simulink model "test_mdl"  (R2018a)
settings: Solver=VariableStepAuto  StartTime=0.0  StopTime=10.0  RelTol=1e-3
(part 6 of 8)

== system test_mdl/FD1_CAN_P702_GASD_MY21_DCV_V06/IPMA_ADAS/PARSEDPhysSODLtoGWM_ECG ==
  PARSEDPhysSODLtoGWM_ECG : Constant
  bus_creator : BusCreator  Inputs=1
  port : Outport
  wires:
  bus_creator/1 -> port/1  "PARSEDPhysSODLtoGWM_ECG"
  PARSEDPhysSODLtoGWM_ECG/1 -> bus_creator/1  "PARSEDPhysSODLtoGWM_ECG"

== system test_mdl/FD1_CAN_P702_GASD_MY21_DCV_V06/IPMA_ADAS/PARSEDPhysSODRtoGWM_ECG ==
  PARSEDPhysSODRtoGWM_ECG : Constant
  bus_creator : BusCreator  Inputs=1
  port : Outport
  wires:
  bus_creator/1 -> port/1  "PARSEDPhysSODRtoGWM_ECG"
  PARSEDPhysSODRtoGWM_ECG/1 -> bus_creator/1  "PARSEDPhysSODRtoGWM_ECG"

== system test_mdl/FD1_CAN_P702_GASD_MY21_DCV_V06/IPMA_ADAS/PARSEDPushCCMtoGWM_ECG ==
  PARSEDPhysCCM2toGWM_ECG : Constant
  bus_creator : BusCreator  Inputs=1
  port : Outport
  wires:
  bus_creator/1 -> port/1  "PARSEDPushCCMtoGWM_ECG"
  PARSEDPhysCCM2toGWM_ECG/1 -> bus_creator/1  "PARSEDPhysCCM2toGWM_ECG"

== system test_mdl/FD1_CAN_P702_GASD_MY21_DCV_V06/IPMA_ADAS/PARSEDPushIPMAtoGWM_ECG ==
  PARSEDPhysIPMA2toGWM_ECG : Constant
  bus_creator : BusCreator  Inputs=1
  port : Outport
  wires:
  bus_creator/1 -> port/1  "PARSEDPushIPMAtoGWM_ECG"
  PARSEDPhysIPMA2toGWM_ECG/1 -> bus_creator/1  "PARSEDPhysIPMA2toGWM_ECG"

== system test_mdl/FD1_CAN_P702_GASD_MY21_DCV_V06/IPMA_ADAS/PARSEDPushSODCMCtoGWM ==
  PARSEDPhysSODCMC2toGWM_ECG : Constant
  bus_creator : BusCreator  Inputs=1
  port : Outport
  wires:
  bus_creator/1 -> port/1  "PARSEDPushSODCMCtoGWM"
  PARSEDPhysSODCMC2toGWM_ECG/1 -> bus_creator/1  "PARSEDPhysSODCMC2toGWM_ECG"

== system test_mdl/FD1_CAN_P702_GASD_MY21_DCV_V06/IPMA_ADAS/PARSEDPushSODCMDtoGWM ==
  PARSEDPhysSODCMD2toGWM_ECG : Constant
  bus_creator : BusCreator  Inputs=1
  port : Outport
  wires:
  bus_creator/1 -> port/1  "PARSEDPushSODCMDtoGWM"
  PARSEDPhysSODCMD2toGWM_ECG/1 -> bus_creator/1  "PARSEDPhysSODCMD2toGWM_ECG"

== system test_mdl/FD1_CAN_P702_GASD_MY21_DCV_V06/IPMA_ADAS/PARSEDPushSODLtoGWM_ECG ==
  PARSEDPhysSODL2toGWM_ECG : Constant
  bus_creator : BusCreator  Inputs=1
  port : Outport
  wires:
  bus_creator/1 -> port/1  "PARSEDPushSODLtoGWM_ECG"
  PARSEDPhysSODL2toGWM_ECG/1 -> bus_creator/1  "PARSEDPhysSODL2toGWM_ECG"

== system test_mdl/FD1_CAN_P702_GASD_MY21_DCV_V06/IPMA_ADAS/PARSEDPushSODRtoGWM_ECG ==
  PARSEDPhysSODR2toGWM_ECG : Constant
  bus_creator : BusCreator  Inputs=1
  port : Outport
  wires:
  bus_creator/1 -> port/1  "PARSEDPushSODRtoGWM_ECG"
  PARSEDPhysSODR2toGWM_ECG/1 -> bus_creator/1  "PARSEDPhysSODR2toGWM_ECG"

== system test_mdl/FD1_CAN_P702_GASD_MY21_DCV_V06/IPMA_ADAS/ParkAid_Aud_Warn_Stat ==
  ApaActvSd_D_Actl : Constant
  ApaMde_D_Avail : Constant
  ApaMde_D_Stat : Constant
  FpaChime_D_Rq : Constant
  PrkAidAudioMute_B_Rq : Constant
  PrkAidMsgTxt_D_Rq : Constant
  PrkAidSnsFlCntr_D_Stat : Constant
  PrkAidSnsFlCrnr_D_Stat : Constant
  PrkAidSnsFrCntr_D_Stat : Constant
  PrkAidSnsFrCrnr_D_Stat : Constant
  PrkAidSwtch_B_Stat : Constant
  PrkBrkEl_B_RqFap : Constant
  RpaChime_D_Rq : Constant
  SidePrkSnsL1_D_Stat : Constant
  SidePrkSnsL2_D_Stat : Constant
  SidePrkSnsR1_D_Stat : Constant
  SidePrkSnsR2_D_Stat : Constant
  bus_creator : BusCreator  Inputs=17
  port : Outport
  wires:
  bus_creator/1 -> port/1  "ParkAid_Aud_Warn_Stat"
  ApaActvSd_D_Actl/1 -> bus_creator/1  "ApaActvSd_D_Actl"
  ApaMde_D_Avail/1 -> bus_creator/2  "ApaMde_D_Avail"
  ApaMde_D_Stat/1 -> bus_creator/3  "ApaMde_D_Stat"
  FpaChime_D_Rq/1 -> bus_creator/4  "FpaChime_D_Rq"
  PrkAidAudioMute_B_Rq/1 -> bus_creator/5  "PrkAidAudioMute_B_Rq"
  PrkAidMsgTxt_D_Rq/1 -> bus_creator/6  "PrkAidMsgTxt_D_Rq"
  PrkAidSnsFlCntr_D_Stat/1 -> bus_creator/7  "PrkAidSnsFlCntr_D_Stat"
  PrkAidSnsFlCrnr_D_Stat/1 -> bus_creator/8  "PrkAidSnsFlCrnr_D_Stat"
  PrkAidSnsFrCntr_D_Stat/1 -> bus_creator/9  "PrkAidSnsFrCntr_D_Stat"
  PrkAidSnsFrCrnr_D_Stat/1 -> bus_creator/10  "PrkAidSnsFrCrnr_D_Stat"
  PrkAidSwtch_B_Stat/1 -> bus_creator/11  "PrkAidSwtch_B_Stat"
  PrkBrkEl_B_RqFap/1 -> bus_creator/12  "PrkBrkEl_B_RqFap"
  RpaChime_D_Rq/1 -> bus_creator/13  "RpaChime_D_Rq"
  SidePrkSnsL1_D_Stat/1 -> bus_creator/14  "SidePrkSnsL1_D_Stat"
  SidePrkSnsL2_D_Stat/1 -> bus_creator/15  "SidePrkSnsL2_D_Stat"
  SidePrkSnsR1_D_Stat/1 -> bus_creator/16  "SidePrkSnsR1_D_Stat"
  SidePrkSnsR2_D_Stat/1 -> bus_creator/17  "SidePrkSnsR2_D_Stat"

== system test_mdl/FD1_CAN_P702_GASD_MY21_DCV_V06/IPMA_ADAS/ParkAid_Aud_Warn_Stat2 ==
  ApaBrk_A_Rq : Constant
  ApaBrk_D_Rq : Constant
  ApaLongCtrlEnbl_D_Rq : Constant
  PrkAidChime_D_Stat : Constant
  PrkAidFront_D_Stat : Constant
  PrkAidLamp_D_Rq : Constant
  PrkAidRear_D_Stat : Constant
  PrkAidSnsRlCntr_D_Stat : Constant
  PrkAidSnsRlCrnr_D_Stat : Constant
  PrkAidSnsRrCntr_D_Stat : Constant
  PrkAidSnsRrCrnr_D_Stat : Constant
  PrkAid_D_Falt : Constant
  SidePrkSnsL3_D_Stat : Constant
  SidePrkSnsL4_D_Stat : Constant
  SidePrkSnsR3_D_Stat : Constant
  SidePrkSnsR4_D_Stat : Constant
  bus_creator : BusCreator  Inputs=16
  port : Outport
  wires:
  bus_creator/1 -> port/1  "ParkAid_Aud_Warn_Stat2"
  ApaBrk_A_Rq/1 -> bus_creator/1  "ApaBrk_A_Rq"
  ApaBrk_D_Rq/1 -> bus_creator/2  "ApaBrk_D_Rq"
  ApaLongCtrlEnbl_D_Rq/1 -> bus_creator/3  "ApaLongCtrlEnbl_D_Rq"
  PrkAidChime_D_Stat/1 -> bus_creator/4  "PrkAidChime_D_Stat"
  PrkAidFront_D_Stat/1 -> bus_creator/5  "PrkAidFront_D_Stat"
  PrkAidLamp_D_Rq/1 -> bus_creator/6  "PrkAidLamp_D_Rq"
  PrkAidRear_D_Stat/1 -> bus_creator/7  "PrkAidRear_D_Stat"
  PrkAidSnsRlCntr_D_Stat/1 -> bus_creator/8  "PrkAidSnsRlCntr_D_Stat"
  PrkAidSnsRlCrnr_D_Stat/1 -> bus_creator/9  "PrkAidSnsRlCrnr_D_Stat"
  PrkAidSnsRrCntr_D_Stat/1 -> bus_creator/10  "PrkAidSnsRrCntr_D_Stat"
  PrkAidSnsRrCrnr_D_Stat/1 -> bus_creator/11  "PrkAidSnsRrCrnr_D_Stat"
  PrkAid_D_Falt/1 -> bus_creator/12  "PrkAid_D_Falt"
  SidePrkSnsL3_D_Stat/1 -> bus_creator/13  "SidePrkSnsL3_D_Stat"
  SidePrkSnsL4_D_Stat/1 -> bus_creator/14  "SidePrkSnsL4_D_Stat"
  SidePrkSnsR3_D_Stat/1 -> bus_creator/15  "SidePrkSnsR3_D_Stat"
  SidePrkSnsR4_D_Stat/1 -> bus_creator/16  "SidePrkSnsR4_D_Stat"

== system test_mdl/FD1_CAN_P702_GASD_MY21_DCV_V06/IPMA_ADAS/ParkAid_Data ==
  ApaAcsy_D_RqDrv : Constant
  ApaActvSide2_D_Stat : Constant
  ApaButtnPrssd_B_Stat : Constant
  ApaChime_D_Rq : Constant
  ApaGearShif_D_RqDrv : Constant
  ApaLongCtl_D_RqDrv : Constant
  ApaMsgTxt_D_Rq : Constant
  ApaScan_D_Stat : Constant
  ApaSelPoa_D_Stat : Constant
  ApaSelPpa_D_Stat : Constant
  ApaSelSapp_D_Stat : Constant
  ApaSteScanMde_D_Stat : Constant
  ApaSteWhl_D_RqDrv : Constant
  ApaSys_D_Stat : Constant
  ApaTrgtDist_D_Stat : Constant
  EPASExtAngleStatReq : Constant
  ExtSteeringAngleReq2 : Constant
  SAPPStatusCoding : Constant
  bus_creator : BusCreator  Inputs=18
  port : Outport
  wires:
  bus_creator/1 -> port/1  "ParkAid_Data"
  ApaAcsy_D_RqDrv/1 -> bus_creator/1  "ApaAcsy_D_RqDrv"
  ApaActvSide2_D_Stat/1 -> bus_creator/2  "ApaActvSide2_D_Stat"
  ApaButtnPrssd_B_Stat/1 -> bus_creator/3  "ApaButtnPrssd_B_Stat"
  ApaChime_D_Rq/1 -> bus_creator/4  "ApaChime_D_Rq"
  ApaGearShif_D_RqDrv/1 -> bus_creator/5  "ApaGearShif_D_RqDrv"
  ApaLongCtl_D_RqDrv/1 -> bus_creator/6  "ApaLongCtl_D_RqDrv"
  ApaMsgTxt_D_Rq/1 -> bus_creator/7  "ApaMsgTxt_D_Rq"
  ApaScan_D_Stat/1 -> bus_creator/8  "ApaScan_D_Stat"
  ApaSelPoa_D_Stat/1 -> bus_creator/9  "ApaSelPoa_D_Stat"
  ApaSelPpa_D_Stat/1 -> bus_creator/10  "ApaSelPpa_D_Stat"
  ApaSelSapp_D_Stat/1 -> bus_creator/11  "ApaSelSapp_D_Stat"
  ApaSteScanMde_D_Stat/1 -> bus_creator/12  "ApaSteScanMde_D_Stat"
  ApaSteWhl_D_RqDrv/1 -> bus_creator/13  "ApaSteWhl_D_RqDrv"
  ApaSys_D_Stat/1 -> bus_creator/14  "ApaSys_D_Stat"
  ApaTrgtDist_D_Stat/1 -> bus_creator/15  "ApaTrgtDist_D_Stat"
  EPASExtAngleStatReq/1 -> bus_creator/16  "EPASExtAngleStatReq"
  ExtSteeringAngleReq2/1 -> bus_creator/17  "ExtSteeringAngleReq2"
  SAPPStatusCoding/1 -> bus_creator/18  "SAPPStatusCoding"

== system test_mdl/FD1_CAN_P702_GASD_MY21_DCV_V06/IPMA_ADAS/ParkAid_Data2 ==
  PrkAidAcsyFront_D_Stat : Constant
  PrkAidAcsyRear_D_Stat : Constant
  PrkAidDrvDir_D_Stat : Constant
  PrkAidRdiusLeft_L_Dsply : Constant
  PrkAidRdiusRight_L_Dsply : Constant
  bus_creator : BusCreator  Inputs=5
  port : Outport
  wires:
  bus_creator/1 -> port/1  "ParkAid_Data2"
  PrkAidAcsyFront_D_Stat/1 -> bus_creator/1  "PrkAidAcsyFront_D_Stat"
  PrkAidAcsyRear_D_Stat/1 -> bus_creator/2  "PrkAidAcsyRear_D_Stat"
  PrkAidDrvDir_D_Stat/1 -> bus_creator/3  "PrkAidDrvDir_D_Stat"
  PrkAidRdiusLeft_L_Dsply/1 -> bus_creator/4  "PrkAidRdiusLeft_L_Dsply"
  PrkAidRdiusRight_L_Dsply/1 -> bus_creator/5  "PrkAidRdiusRight_L_Dsply"

== system test_mdl/FD1_CAN_P702_GASD_MY21_DCV_V06/IPMA_ADAS/ParkAid_Data_2 ==
  FapLcDistToObj_L_Actl : Constant
  TrnRngDRqFap_No_Cnt : Constant
  TrnRngDRqFap_No_Cs : Constant
  TrnRng_D_RqFap : Constant
  Veh_V_RqFap : Constant
  bus_creator : BusCreator  Inputs=5
  port : Outport
  wires:
  bus_creator/1 -> port/1  "ParkAid_Data_2"
  FapLcDistToObj_L_Actl/1 -> bus_creator/1  "FapLcDistToObj_L_Actl"
  TrnRngDRqFap_No_Cnt/1 -> bus_creator/2  "TrnRngDRqFap_No_Cnt"
  TrnRngDRqFap_No_Cs/1 -> bus_creator/3  "TrnRngDRqFap_No_Cs"
  TrnRng_D_RqFap/1 -> bus_creator/4  "TrnRng_D_RqFap"
  Veh_V_RqFap/1 -> bus_creator/5  "Veh_V_RqFap"

== system test_mdl/FD1_CAN_P702_GASD_MY21_DCV_V06/IPMA_ADAS/Personality_CCM_Data ==
  FeatConfigCcmActl : Constant
  FeatNoCcmActl : Constant
  PersIndexCcm_D_Actl : Constant
  bus_creator : BusCreator  Inputs=3
  port : Outport
  wires:
  bus_creator/1 -> port/1  "Personality_CCM_Data"
  FeatConfigCcmActl/1 -> bus_creator/1  "FeatConfigCcmActl"
  FeatNoCcmActl/1 -> bus_creator/2  "FeatNoCcmActl"
  PersIndexCcm_D_Actl/1 -> bus_creator/3  "PersIndexCcm_D_Actl"

== system test_mdl/FD1_CAN_P702_GASD_MY21_DCV_V06/IPMA_ADAS/Personality_IPMB_Data ==
  FeatConfigIpmbActl : Constant
  FeatNoIpmbActl : Constant
  PersIndexIpmb_D_Actl : Constant
  bus_creator : BusCreator  Inputs=3
  port : Outport
  wires:
  bus_creator/1 -> port/1  "Personality_IPMB_Data"
  FeatConfigIpmbActl/1 -> bus_creator/1  "FeatConfigIpmbActl"
  FeatNoIpmbActl/1 -> bus_creator/2  "FeatNoIpmbActl"
  PersIndexIpmb_D_Actl/1 -> bus_creator/3  "PersIndexIpmb_D_Actl"

== system test_mdl/FD1_CAN_P702_GASD_MY21_DCV_V06/IPMA_ADAS/Side_Detect_L_Stat ==
  BttLeft_D_RqDrv : Constant
  BttLeft_D_Stat : Constant
  CtaAlrtLeft2_D_Stat : Constant
  CtaAlrtLeft_D_Stat : Constant
  CtaBrkLeftMsgTxt_B_Rq : Constant
  CtaLeftBrkDecel_B_Rq : Constant
  CtaLeftBrkEnbl_B_Rq : Constant
  CtaLeft_D_Stat : Constant
  CtaSnsLeft_D_Stat : Constant
  Side_Detect_L_Illum : Constant
  SodAlrtLeft_D_Stat : Constant
  SodDetctLeft_D_Stat : Constant
  SodLeft_D_Stat : Constant
  SodSnsLeft_D_Stat : Constant
  SodWarnLeft_Prd_Rq : Constant
  bus_creator : BusCreator  Inputs=15
  port : Outport
  wires:
  bus_creator/1 -> port/1  "Side_Detect_L_Stat"
  BttLeft_D_RqDrv/1 -> bus_creator/1  "BttLeft_D_RqDrv"
  BttLeft_D_Stat/1 -> bus_creator/2  "BttLeft_D_Stat"
  CtaAlrtLeft2_D_Stat/1 -> bus_creator/3  "CtaAlrtLeft2_D_Stat"
  CtaAlrtLeft_D_Stat/1 -> bus_creator/4  "CtaAlrtLeft_D_Stat"
  CtaBrkLeftMsgTxt_B_Rq/1 -> bus_creator/5  "CtaBrkLeftMsgTxt_B_Rq"
  CtaLeftBrkDecel_B_Rq/1 -> bus_creator/6  "CtaLeftBrkDecel_B_Rq"
  CtaLeftBrkEnbl_B_Rq/1 -> bus_creator/7  "CtaLeftBrkEnbl_B_Rq"
  CtaLeft_D_Stat/1 -> bus_creator/8  "CtaLeft_D_Stat"
  CtaSnsLeft_D_Stat/1 -> bus_creator/9  "CtaSnsLeft_D_Stat"
  Side_Detect_L_Illum/1 -> bus_creator/10  "Side_Detect_L_Illum"
  SodAlrtLeft_D_Stat/1 -> bus_creator/11  "SodAlrtLeft_D_Stat"
  SodDetctLeft_D_Stat/1 -> bus_creator/12  "SodDetctLeft_D_Stat"
  SodLeft_D_Stat/1 -> bus_creator/13  "SodLeft_D_Stat"
  SodSnsLeft_D_Stat/1 -> bus_creator/14  "SodSnsLeft_D_Stat"
  SodWarnLeft_Prd_Rq/1 -> bus_creator/15  "SodWarnLeft_Prd_Rq"

== system test_mdl/FD1_CAN_P702_GASD_MY21_DCV_V06/IPMA_ADAS/Side_Detect_R_Stat ==
  BttRight_D_RqDrv : Constant
  BttRight_D_Stat : Constant
  CtaAlrtRight2_D_Stat : Constant
  CtaAlrtRight_D_Stat : Constant
  CtaBrkRightMsgTxt_B_Rq : Constant
  CtaRightBrkDecel_B_Rq : Constant
  CtaRightBrkEnbl_B_Rq : Constant
  CtaRight_D_Stat : Constant
  CtaSnsRight_D_Stat : Constant
  Side_Detect_R_Illum : Constant
  SodAlrtRight_D_Stat : Constant
  SodDetctRight_D_Stat : Constant
  SodRight_D_Stat : Constant
  SodSnsRight_D_Stat : Constant
  SodWarnRight_Prd_Rq : Constant
  bus_creator : BusCreator  Inputs=15
  port : Outport
  wires:
  bus_creator/1 -> port/1  "Side_Detect_R_Stat"
  BttRight_D_RqDrv/1 -> bus_creator/1  "BttRight_D_RqDrv"
  BttRight_D_Stat/1 -> bus_creator/2  "BttRight_D_Stat"
  CtaAlrtRight2_D_Stat/1 -> bus_creator/3  "CtaAlrtRight2_D_Stat"
  CtaAlrtRight_D_Stat/1 -> bus_creator/4  "CtaAlrtRight_D_Stat"
  CtaBrkRightMsgTxt_B_Rq/1 -> bus_creator/5  "CtaBrkRightMsgTxt_B_Rq"
  CtaRightBrkDecel_B_Rq/1 -> bus_creator/6  "CtaRightBrkDecel_B_Rq"
  CtaRightBrkEnbl_B_Rq/1 -> bus_creator/7  "CtaRightBrkEnbl_B_Rq"
  CtaRight_D_Stat/1 -> bus_creator/8  "CtaRight_D_Stat"
  CtaSnsRight_D_Stat/1 -> bus_creator/9  "CtaSnsRight_D_Stat"
  Side_Detect_R_Illum/1 -> bus_creator/10  "Side_Detect_R_Illum"
  SodAlrtRight_D_Stat/1 -> bus_creator/11  "SodAlrtRight_D_Stat"
  SodDetctRight_D_Stat/1 -> bus_creator/12  "SodDetctRight_D_Stat"
  SodRight_D_Stat/1 -> bus_creator/13  "SodRight_D_Stat"
  SodSnsRight_D_Stat/1 -> bus_creator/14  "SodSnsRight_D_Stat"
  SodWarnRight_Prd_Rq/1 -> bus_creator/15  "SodWarnRight_Prd_Rq"

== system test_mdl/FD1_CAN_P702_GASD_MY21_DCV_V06/IPMA_ADAS/Steer_Assist_Data ==
  CmbbObjClass_D_Stat : Constant
  CmbbObjColl_T_Actl : Constant
  CmbbObjConfdnc_D_Stat : Constant
  CmbbObjDistLat_L_Actl : Constant
  CmbbObjDistLong_L_Actl : Constant
  CmbbObjRelLat_V_Actl : Constant
  CmbbObjRelLong_V_Actl : Constant
  EsaEnbl_D2_Rq : Constant
  bus_creator : BusCreator  Inputs=8
  port : Outport
  wires:
  bus_creator/1 -> port/1  "Steer_Assist_Data"
  CmbbObjClass_D_Stat/1 -> bus_creator/1  "CmbbObjClass_D_Stat"
  CmbbObjColl_T_Actl/1 -> bus_creator/2  "CmbbObjColl_T_Actl"
  CmbbObjConfdnc_D_Stat/1 -> bus_creator/3  "CmbbObjConfdnc_D_Stat"
  CmbbObjDistLat_L_Actl/1 -> bus_creator/4  "CmbbObjDistLat_L_Actl"
  CmbbObjDistLong_L_Actl/1 -> bus_creator/5  "CmbbObjDistLong_L_Actl"
  CmbbObjRelLat_V_Actl/1 -> bus_creator/6  "CmbbObjRelLat_V_Actl"
  CmbbObjRelLong_V_Actl/1 -> bus_creator/7  "CmbbObjRelLong_V_Actl"
  EsaEnbl_D2_Rq/1 -> bus_creator/8  "EsaEnbl_D2_Rq"

== system test_mdl/FD1_CAN_P702_GASD_MY21_DCV_V06/IPMA_ADAS/SuspensionRoad_Data ==
  SrpDistLeft_L_Actl : Constant
  SrpDistRight_L_Actl : Constant
  SrpEventLeft_D_Stat : Constant
  SrpEventRight_D_Stat : Constant
  SrpHghtLeft_L_Actl : Constant
  SrpHghtRight_L_Actl : Constant
  SrpSigValid_B_Stat : Constant
  SuspClkSync_No_Actl : Constant
  bus_creator : BusCreator  Inputs=8
  port : Outport
  wires:
  bus_creator/1 -> port/1  "SuspensionRoad_Data"
  SrpDistLeft_L_Actl/1 -> bus_creator/1  "SrpDistLeft_L_Actl"
  SrpDistRight_L_Actl/1 -> bus_creator/2  "SrpDistRight_L_Actl"
  SrpEventLeft_D_Stat/1 -> bus_creator/3  "SrpEventLeft_D_Stat"
  SrpEventRight_D_Stat/1 -> bus_creator/4  "SrpEventRight_D_Stat"
  SrpHghtLeft_L_Actl/1 -> bus_creator/5  "SrpHghtLeft_L_Actl"
  SrpHghtRight_L_Actl/1 -> bus_creator/6  "SrpHghtRight_L_Actl"
  SrpSigValid_B_Stat/1 -> bus_creator/7  "SrpSigValid_B_Stat"
  SuspClkSync_No_Actl/1 -> bus_creator/8  "SuspClkSync_No_Actl"

== system test_mdl/FD1_CAN_P702_GASD_MY21_DCV_V06/IPMA_ADAS/TesterPhysicalResCCM ==
  TesterPhysicalResCCM : Constant
  bus_creator : BusCreator  Inputs=1
  port : Outport
  wires:
  bus_creator/1 -> port/1  "TesterPhysicalResCCM"
  TesterPhysicalResCCM/1 -> bus_creator/1  "TesterPhysicalResCCM"

== system test_mdl/FD1_CAN_P702_GASD_MY21_DCV_V06/IPMA_ADAS/TesterPhysicalResIPMA ==
  TesterPhysicalResIPMA : Constant
  bus_creator : BusCreator  Inputs=1
  port : Outport
  wires:
  bus_creator/1 -> port/1  "TesterPhysicalResIPMA"
  TesterPhysicalResIPMA/1 -> bus_creator/1  "TesterPhysicalResIPMA"

== system test_mdl/FD1_CAN_P702_GASD_MY21_DCV_V06/IPMA_ADAS/TesterPhysicalResSODCMC ==
  TesterPhysicalResSODCMC : Constant
  bus_creator : BusCreator  Inputs=1
  port : Outport
  wires:
  bus_creator/1 -> port/1  "TesterPhysicalResSODCMC"
  TesterPhysicalResSODCMC/1 -> bus_creator/1  "TesterPhysicalResSODCMC"

== system test_mdl/FD1_CAN_P702_GASD_MY21_DCV_V06/IPMA_ADAS/TesterPhysicalResSODCMD ==
  TesterPhysicalResSODCMD : Constant
  bus_creator : BusCreator  Inputs=1
  port : Outport
  wires:
  bus_creator/1 -> port/1  "TesterPhysicalResSODCMD"
  TesterPhysicalResSODCMD/1 -> bus_creator/1  "TesterPhysicalResSODCMD"

== system test_mdl/FD1_CAN_P702_GASD_MY21_DCV_V06/IPMA_ADAS/TesterPhysicalResSODL ==
  TesterPhysicalResSODL : Constant
  bus_creator : BusCreator  Inputs=1
  port : Outport
  wires:
  bus_creator/1 -> port/1  "TesterPhysicalResSODL"
  TesterPhysicalResSODL/1 -> bus_creator/1  "TesterPhysicalResSODL"

== system test_mdl/FD1_CAN_P702_GASD_MY21_DCV_V06/IPMA_ADAS/TesterPhysicalResSODR ==
  TesterPhysicalResSODR : Constant
  bus_creator : BusCreator  Inputs=1
  port : Outport
  wires:
  bus_creator/1 -> port/1  "TesterPhysicalResSODR"
  TesterPhysicalResSODR/1 -> bus_creator/1  "TesterPhysicalResSODR"

== system test_mdl/FD1_CAN_P702_GASD_MY21_DCV_V06/IPMA_ADAS/Traffic_RecognitnData ==
  TsrMsgTxt_D_Rq : Constant
  TsrOswWarnMsgTxt_D_Rq : Constant
  TsrOvtkMsgTxt2_D_Rq : Constant
  TsrOvtkMsgTxt_D_Rq : Constant
  TsrOvtkStatMsgTxt_D_Rq : Constant
  TsrStatMsgTxt_D_Rq : Constant
  TsrVLim1MsgTxt_D_Rq : Constant
  TsrVLim2MsgTxt_D_Rq : Constant
  TsrVl1PrmntMsgTxt_D_Rq : Constant
  TsrVl1RstrcMsgTxt2_D_Rq : Constant
  TsrVl1RstrcMsgTxt_D_Rq : Constant
  TsrVl1StatMsgTxt_D_Rq : Constant
  TsrVl2PrmntMsgTxt_D_Rq : Constant
  TsrVl2RstrcMsgTxt2_D_Rq : Constant
  TsrVl2RstrcMsgTxt_D_Rq : Constant
  TsrVl2StatMsgTxt_D_Rq : Constant
  TsrVlUnitMsgTxt_D_Rq : Constant
  WwaWarn_B_Rq : Constant
  bus_creator : BusCreator  Inputs=18
  port : Outport
  wires:
  bus_creator/1 -> port/1  "Traffic_RecognitnData"
  TsrMsgTxt_D_Rq/1 -> bus_creator/1  "TsrMsgTxt_D_Rq"
  TsrOswWarnMsgTxt_D_Rq/1 -> bus_creator/2  "TsrOswWarnMsgTxt_D_Rq"
  TsrOvtkMsgTxt2_D_Rq/1 -> bus_creator/3  "TsrOvtkMsgTxt2_D_Rq"
  TsrOvtkMsgTxt_D_Rq/1 -> bus_creator/4  "TsrOvtkMsgTxt_D_Rq"
  TsrOvtkStatMsgTxt_D_Rq/1 -> bus_creator/5  "TsrOvtkStatMsgTxt_D_Rq"
  TsrStatMsgTxt_D_Rq/1 -> bus_creator/6  "TsrStatMsgTxt_D_Rq"
  TsrVLim1MsgTxt_D_Rq/1 -> bus_creator/7  "TsrVLim1MsgTxt_D_Rq"
  TsrVLim2MsgTxt_D_Rq/1 -> bus_creator/8  "TsrVLim2MsgTxt_D_Rq"
  TsrVl1PrmntMsgTxt_D_Rq/1 -> bus_creator/9  "TsrVl1PrmntMsgTxt_D_Rq"
  TsrVl1RstrcMsgTxt2_D_Rq/1 -> bus_creator/10  "TsrVl1RstrcMsgTxt2_D_Rq"
  TsrVl1RstrcMsgTxt_D_Rq/1 -> bus_creator/11  "TsrVl1RstrcMsgTxt_D_Rq"
  TsrVl1StatMsgTxt_D_Rq/1 -> bus_creator/12  "TsrVl1StatMsgTxt_D_Rq"
  TsrVl2PrmntMsgTxt_D_Rq/1 -> bus_creator/13  "TsrVl2PrmntMsgTxt_D_Rq"
  TsrVl2RstrcMsgTxt2_D_Rq/1 -> bus_creator/14  "TsrVl2RstrcMsgTxt2_D_Rq"
  TsrVl2RstrcMsgTxt_D_Rq/1 -> bus_creator/15  "TsrVl2RstrcMsgTxt_D_Rq"
  TsrVl2StatMsgTxt_D_Rq/1 -> bus_creator/16  "TsrVl2StatMsgTxt_D_Rq"
  TsrVlUnitMsgTxt_D_Rq/1 -> bus_creator/17  "TsrVlUnitMsgTxt_D_Rq"
  WwaWarn_B_Rq/1 -> bus_creator/18  "WwaWarn_B_Rq"

== system test_mdl/FD1_CAN_P702_GASD_MY21_DCV_V06/IPMA_ADAS/TrailerAid_Stat3 ==
  HitchToTrlrAxle_L_Calc2 : Constant
  HitchToVehAxle_L_Calc : Constant
  TrlrAidTrgtId_No_Actl : Constant
  TrlrAid_An3_Actl : Constant
  TrlrAid_AnRate2_Actl : Constant
  TrlrAid_D2_Stat : Constant
  TrlrAnCalib_B_Complt : Constant
  TrlrAnOffstDir_D_Calc : Constant
  TrlrAnOffst_An_Calc : Constant
  TrlrRvrse_D_Stat : Constant
  TrlrTrgtAcquire_D_Stat : Constant
  bus_creator : BusCreator  Inputs=11
  port : Outport
  wires:
  bus_creator/1 -> port/1  "TrailerAid_Stat3"
  HitchToTrlrAxle_L_Calc2/1 -> bus_creator/1  "HitchToTrlrAxle_L_Calc2"
  HitchToVehAxle_L_Calc/1 -> bus_creator/2  "HitchToVehAxle_L_Calc"
  TrlrAidTrgtId_No_Actl/1 -> bus_creator/3  "TrlrAidTrgtId_No_Actl"
  TrlrAid_An3_Actl/1 -> bus_creator/4  "TrlrAid_An3_Actl"
  TrlrAid_AnRate2_Actl/1 -> bus_creator/5  "TrlrAid_AnRate2_Actl"
  TrlrAid_D2_Stat/1 -> bus_creator/6  "TrlrAid_D2_Stat"
  TrlrAnCalib_B_Complt/1 -> bus_creator/7  "TrlrAnCalib_B_Complt"
  TrlrAnOffstDir_D_Calc/1 -> bus_creator/8  "TrlrAnOffstDir_D_Calc"
  TrlrAnOffst_An_Calc/1 -> bus_creator/9  "TrlrAnOffst_An_Calc"
  TrlrRvrse_D_Stat/1 -> bus_creator/10  "TrlrRvrse_D_Stat"
  TrlrTrgtAcquire_D_Stat/1 -> bus_creator/11  "TrlrTrgtAcquire_D_Stat"

== system test_mdl/FD1_CAN_P702_GASD_MY21_DCV_V06/PCM/DCACA_Data4 ==
  DcacElPw_D_Stat : Constant
  DcacEngOnMsgTxt_D_Rq : Constant
  DcacFaltMsgTxt_D_Rq : Constant
  DcacGfciTest_B_Rq : Constant
  DcacHw_D_Confg : Constant
  DcacLedCtl_D_Rq : Constant
  DcacLoFuelMsgTxt_D_Rq : Constant
  DcacOn_B_Rq : Constant
  DcacOut1_Pw_Dsply : Constant
  DcacOut2_Pw_Dsply : Constant
  DcacOut_Pw_DsplyMx : Constant
  DcacSys_B_Falt : Constant
  PwBedPnlEnbl_B_Rq : Constant
  bus_creator : BusCreator  Inputs=13
  port : Outport
  wires:
  bus_creator/1 -> port/1  "DCACA_Data4"
  DcacElPw_D_Stat/1 -> bus_creator/1  "DcacElPw_D_Stat"
  DcacEngOnMsgTxt_D_Rq/1 -> bus_creator/2  "DcacEngOnMsgTxt_D_Rq"
  DcacFaltMsgTxt_D_Rq/1 -> bus_creator/3  "DcacFaltMsgTxt_D_Rq"
  DcacGfciTest_B_Rq/1 -> bus_creator/4  "DcacGfciTest_B_Rq"
  DcacHw_D_Confg/1 -> bus_creator/5  "DcacHw_D_Confg"
  DcacLedCtl_D_Rq/1 -> bus_creator/6  "DcacLedCtl_D_Rq"
  DcacLoFuelMsgTxt_D_Rq/1 -> bus_creator/7  "DcacLoFuelMsgTxt_D_Rq"
  DcacOn_B_Rq/1 -> bus_creator/8  "DcacOn_B_Rq"
  DcacOut1_Pw_Dsply/1 -> bus_creator/9  "DcacOut1_Pw_Dsply"
  DcacOut2_Pw_Dsply/1 -> bus_creator/10  "DcacOut2_Pw_Dsply"
  DcacOut_Pw_DsplyMx/1 -> bus_creator/11  "DcacOut_Pw_DsplyMx"
  DcacSys_B_Falt/1 -> bus_creator/12  "DcacSys_B_Falt"
  PwBedPnlEnbl_B_Rq/1 -> bus_creator/13  "PwBedPnlEnbl_B_Rq"

== system test_mdl/FD1_CAN_P702_GASD_MY21_DCV_V06/PCM/EngBrakeData ==
  AccEngStat_D_Actl : Constant
  AccStopMde_D_Rq : Constant
  BPedDrvAppl_D_QF : Constant
  BpedDrvAppl_D_Actl : Constant
  CcMde_D_Actl : Constant
  CcOvrrdActv_B_Actl : Constant
  CcStat_D_Actl : Constant
  CmbbDeny_B_ActlPrpl : Constant
  CmbbEngTqMn_B_Actl : Constant
  EngAout_N_MnAllw : Constant
  PrplTqMnSat_B_Actl : Constant
  Veh_V_DsplyCcSet : Constant
  bus_creator : BusCreator  Inputs=12
  port : Outport
  wires:
  bus_creator/1 -> port/1  "EngBrakeData"
  AccEngStat_D_Actl/1 -> bus_creator/1  "AccEngStat_D_Actl"
  AccStopMde_D_Rq/1 -> bus_creator/2  "AccStopMde_D_Rq"
  BPedDrvAppl_D_QF/1 -> bus_creator/3  "BPedDrvAppl_D_QF"
  BpedDrvAppl_D_Actl/1 -> bus_creator/4  "BpedDrvAppl_D_Actl"
  CcMde_D_Actl/1 -> bus_creator/5  "CcMde_D_Actl"
  CcOvrrdActv_B_Actl/1 -> bus_creator/6  "CcOvrrdActv_B_Actl"
  CcStat_D_Actl/1 -> bus_creator/7  "CcStat_D_Actl"
  CmbbDeny_B_ActlPrpl/1 -> bus_creator/8  "CmbbDeny_B_ActlPrpl"
  CmbbEngTqMn_B_Actl/1 -> bus_creator/9  "CmbbEngTqMn_B_Actl"
  EngAout_N_MnAllw/1 -> bus_creator/10  "EngAout_N_MnAllw"
  PrplTqMnSat_B_Actl/1 -> bus_creator/11  "PrplTqMnSat_B_Actl"
  Veh_V_DsplyCcSet/1 -> bus_creator/12  "Veh_V_DsplyCcSet"

== system test_mdl/FD1_CAN_P702_GASD_MY21_DCV_V06/PCM/EngVehicleSpThrottle ==
  ApedPosPcActl_D_Qf : Constant
  ApedPosPcActl_No_Cnt : Constant
  ApedPosPcActl_No_Cs : Constant
  ApedPos_PcRate_ActlArb : Constant
  ApedPos_Pc_ActlArb : Constant
  EngAout3_N_Actl : Constant
  EngAoutNActl_D_QF : Constant
  EngAout_N_Actl : Constant
  bus_creator : BusCreator  Inputs=8
  port : Outport
  wires:
  bus_creator/1 -> port/1  "EngVehicleSpThrottle"
  ApedPosPcActl_D_Qf/1 -> bus_creator/1  "ApedPosPcActl_D_Qf"
  ApedPosPcActl_No_Cnt/1 -> bus_creator/2  "ApedPosPcActl_No_Cnt"
  ApedPosPcActl_No_Cs/1 -> bus_creator/3  "ApedPosPcActl_No_Cs"
  ApedPos_PcRate_ActlArb/1 -> bus_creator/4  "ApedPos_PcRate_ActlArb"
  ApedPos_Pc_ActlArb/1 -> bus_creator/5  "ApedPos_Pc_ActlArb"
  EngAout3_N_Actl/1 -> bus_creator/6  "EngAout3_N_Actl"
  EngAoutNActl_D_QF/1 -> bus_creator/7  "EngAoutNActl_D_QF"
  EngAout_N_Actl/1 -> bus_creator/8  "EngAout_N_Actl"

== system test_mdl/FD1_CAN_P702_GASD_MY21_DCV_V06/PCM/EngVehicleSpThrottle2 ==
  GearRvrse_D_Actl : Constant
  StrtrMtrCtlMsgTxt_D2_Rq : Constant
  StrtrMtrCtlMsgTxt_D_Rq : Constant
  StrtrMtrDlyStrt_B_Stat : Constant
  VehVActlEng_D_Qf : Constant
  VehVActlEng_No_Cnt : Constant
  VehVActlEng_No_Cs : Constant
  VehVTrlrAid_B_Avail : Constant
  Veh_V_ActlEng : Constant
  Veh_V_RqCcSet : Constant
  bus_creator : BusCreator  Inputs=10
  port : Outport
  wires:
  bus_creator/1 -> port/1  "EngVehicleSpThrottle2"
  GearRvrse_D_Actl/1 -> bus_creator/1  "GearRvrse_D_Actl"
  StrtrMtrCtlMsgTxt_D2_Rq/1 -> bus_creator/2  "StrtrMtrCtlMsgTxt_D2_Rq"
  StrtrMtrCtlMsgTxt_D_Rq/1 -> bus_creator/3  "StrtrMtrCtlMsgTxt_D_Rq"
  StrtrMtrDlyStrt_B_Stat/1 -> bus_creator/4  "StrtrMtrDlyStrt_B_Stat"
  VehVActlEng_D_Qf/1 -> bus_creator/5  "VehVActlEng_D_Qf"
  VehVActlEng_No_Cnt/1 -> bus_creator/6  "VehVActlEng_No_Cnt"
  VehVActlEng_No_Cs/1 -> bus_creator/7  "VehVActlEng_No_Cs"
  VehVTrlrAid_B_Avail/1 -> bus_creator/8  "VehVTrlrAid_B_Avail"
  Veh_V_ActlEng/1 -> bus_creator/9  "Veh_V_ActlEng"
  Veh_V_RqCcSet/1 -> bus_creator/10  "Veh_V_RqCcSet"

== system test_mdl/FD1_CAN_P702_GASD_MY21_DCV_V06/PCM/EngineClimateData ==
  AirAmbTe_D_Qf : Constant
  AirAmb_P_Actl : Constant
  AirAmb_Te_Actl : Constant
  AirAmb_Te_ActlFilt : Constant
  AslChime_B_Rq : Constant
  AslIconDsply_D_Rq : Constant
  DynoMde_B_Cmd : Constant
  EcssLamp_D_RqDsply : Constant
  EngAout_Aa_Actl : Constant
  GasPrtc_D_RqDsply : Constant
  HvacHtrCore2_Te_Actl : Constant
  bus_creator : BusCreator  Inputs=11
  port : Outport
  wires:
  bus_creator/1 -> port/1  "EngineClimateData"
  AirAmbTe_D_Qf/1 -> bus_creator/1  "AirAmbTe_D_Qf"
  AirAmb_P_Actl/1 -> bus_creator/2  "AirAmb_P_Actl"
  AirAmb_Te_Actl/1 -> bus_creator/3  "AirAmb_Te_Actl"
  AirAmb_Te_ActlFilt/1 -> bus_creator/4  "AirAmb_Te_ActlFilt"
  AslChime_B_Rq/1 -> bus_creator/5  "AslChime_B_Rq"
  AslIconDsply_D_Rq/1 -> bus_creator/6  "AslIconDsply_D_Rq"
  DynoMde_B_Cmd/1 -> bus_creator/7  "DynoMde_B_Cmd"
  EcssLamp_D_RqDsply/1 -> bus_creator/8  "EcssLamp_D_RqDsply"
  EngAout_Aa_Actl/1 -> bus_creator/9  "EngAout_Aa_Actl"
  GasPrtc_D_RqDsply/1 -> bus_creator/10  "GasPrtc_D_RqDsply"
  HvacHtrCore2_Te_Actl/1 -> bus_creator/11  "HvacHtrCore2_Te_Actl"

== system test_mdl/FD1_CAN_P702_GASD_MY21_DCV_V06/PCM/EngineData_1 ==
  SeatWorkSrfc_B_Falt : Constant
  TrnIpcDsplyGear_D_Actl : Constant
  TrnIpcDsplyGear_D_Stat : Constant
  TrnIpcDsplyMde_D_Actl : Constant
  TrnIpcDsplyMde_D_Stat : Constant
  TrnIpcDsplyRng2_D_Actl : Constant
  TrnIpcDsplyRng_D_Stat : Constant
  bus_creator : BusCreator  Inputs=7
  port : Outport
  wires:
  bus_creator/1 -> port/1  "EngineData_1"
  SeatWorkSrfc_B_Falt/1 -> bus_creator/1  "SeatWorkSrfc_B_Falt"
  TrnIpcDsplyGear_D_Actl/1 -> bus_creator/2  "TrnIpcDsplyGear_D_Actl"
  TrnIpcDsplyGear_D_Stat/1 -> bus_creator/3  "TrnIpcDsplyGear_D_Stat"
  TrnIpcDsplyMde_D_Actl/1 -> bus_creator/4  "TrnIpcDsplyMde_D_Actl"
  TrnIpcDsplyMde_D_Stat/1 -> bus_creator/5  "TrnIpcDsplyMde_D_Stat"
  TrnIpcDsplyRng2_D_Actl/1 -> bus_creator/6  "TrnIpcDsplyRng2_D_Actl"
  TrnIpcDsplyRng_D_Stat/1 -> bus_creator/7  "TrnIpcDsplyRng_D_Stat"

== system test_mdl/FD1_CAN_P702_GASD_MY21_DCV_V06/PCM/EngineData_16 ==
  EngAout_N_MxAllw : Constant
  EngExhBrkAutoLamp_B_Rq : Constant
  EngExhBrkMde_D_Actl : Constant
  EngExhBrkOnLamp_B_Rq : Constant
  EngOilLvlWarn_D_Rq1 : Constant
  bus_creator : BusCreator  Inputs=5
  port : Outport
  wires:
  bus_creator/1 -> port/1  "EngineData_16"
  EngAout_N_MxAllw/1 -> bus_creator/1  "EngAout_N_MxAllw"
  EngExhBrkAutoLamp_B_Rq/1 -> bus_creator/2  "EngExhBrkAutoLamp_B_Rq"
  EngExhBrkMde_D_Actl/1 -> bus_creator/3  "EngExhBrkMde_D_Actl"
  EngExhBrkOnLamp_B_Rq/1 -> bus_creator/4  "EngExhBrkOnLamp_B_Rq"
  EngOilLvlWarn_D_Rq1/1 -> bus_creator/5  "EngOilLvlWarn_D_Rq1"

== system test_mdl/FD1_CAN_P702_GASD_MY21_DCV_V06/PCM/EngineData_6 ==
  EngClntTe_D_Qf : Constant
  EngClnt_Te_Actl : Constant
  EngGoutLss_Tq_Est : Constant
  EngOil_Te_Actl : Constant
  EngOvrhtMitgActv_D_Ind : Constant
  bus_creator : BusCreator  Inputs=5
  port : Outport
  wires:
  bus_creator/1 -> port/1  "EngineData_6"
  EngClntTe_D_Qf/1 -> bus_creator/1  "EngClntTe_D_Qf"
  EngClnt_Te_Actl/1 -> bus_creator/2  "EngClnt_Te_Actl"
  EngGoutLss_Tq_Est/1 -> bus_creator/3  "EngGoutLss_Tq_Est"
  EngOil_Te_Actl/1 -> bus_creator/4  "EngOil_Te_Actl"
  EngOvrhtMitgActv_D_Ind/1 -> bus_creator/5  "EngOvrhtMitgActv_D_Ind"

== system test_mdl/FD1_CAN_P702_GASD_MY21_DCV_V06/PCM/EngineData_7 ==
  AirCondClutch_B_Stats : Constant
  AirCondRec_B_Rq : Constant
  EngOilLife_Pc_Actl : Constant
  EngSrvcRqd_B_Rq : Constant
  FuelFillInlet_B_Dsply : Constant
  FuelFilterLamp_B_Dsply : Constant
  FuelFlw_Vl_Dsply : Constant
  HvacAirFullOut_B_Rq : Constant
  OdoCount : Constant
  bus_creator : BusCreator  Inputs=9
  port : Outport
  wires:
  bus_creator/1 -> port/1  "EngineData_7"
  AirCondClutch_B_Stats/1 -> bus_creator/1  "AirCondClutch_B_Stats"
  AirCondRec_B_Rq/1 -> bus_creator/2  "AirCondRec_B_Rq"
  EngOilLife_Pc_Actl/1 -> bus_creator/3  "EngOilLife_Pc_Actl"
  EngSrvcRqd_B_Rq/1 -> bus_creator/4  "EngSrvcRqd_B_Rq"
  FuelFillInlet_B_Dsply/1 -> bus_creator/5  "FuelFillInlet_B_Dsply"
  FuelFilterLamp_B_Dsply/1 -> bus_creator/6  "FuelFilterLamp_B_Dsply"
  FuelFlw_Vl_Dsply/1 -> bus_creator/7  "FuelFlw_Vl_Dsply"
  HvacAirFullOut_B_Rq/1 -> bus_creator/8  "HvacAirFullOut_B_Rq"
  OdoCount/1 -> bus_creator/9  "OdoCount"

== system test_mdl/FD1_CAN_P702_GASD_MY21_DCV_V06/PCM/Engine_Clutch_Data ==
  CluPdlPosPcMeas_D_Qf : Constant
  CluPdlPos_Pc_Meas : Constant
  CluPdl_PcRate_Actl : Constant
  EngAoutIdl_N_Ntrl : Constant
  EngAout_N_Dsply : Constant
  bus_creator : BusCreator  Inputs=5
  port : Outport
  wires:
  bus_creator/1 -> port/1  "Engine_Clutch_Data"
  CluPdlPosPcMeas_D_Qf/1 -> bus_creator/1  "CluPdlPosPcMeas_D_Qf"
  CluPdlPos_Pc_Meas/1 -> bus_creator/2  "CluPdlPos_Pc_Meas"
  CluPdl_PcRate_Actl/1 -> bus_creator/3  "CluPdl_PcRate_Actl"
  EngAoutIdl_N_Ntrl/1 -> bus_creator/4  "EngAoutIdl_N_Ntrl"
  EngAout_N_Dsply/1 -> bus_creator/5  "EngAout_N_Dsply"

== system test_mdl/FD1_CAN_P702_GASD_MY21_DCV_V06/PCM/Gear_Shift_by_Wire_3 ==
  GearSelLck_D_Rq : Constant
  PrkBrkActv_D_RqTrnGear : Constant
  TrnCmdCnt_B_Actl : Constant
  TrnCmdState_B_Actl : Constant
  TrnDtpCmd_D_Actl : Constant
  TrnGearCmd_No_Cnt : Constant
  TrnGearCmd_No_Cs : Constant
  TrnGearCmd_Pc_ActlPt : Constant
  TrnGearMsgTxt_D_Rq : Constant
  TrnGearNtmAllow_B_Stat : Constant
  TrnGear_D_RqPt : Constant
  TrnLvrV_D_Rq : Constant
  TrnNtrlTowCmd_D_Actl : Constant
  TrnSbwSysHlth_D_Actl : Constant
  TrnValidGear_D_Cnfm : Constant
  bus_creator : BusCreator  Inputs=15
  port : Outport
  wires:
  bus_creator/1 -> port/1  "Gear_Shift_by_Wire_3"
  GearSelLck_D_Rq/1 -> bus_creator/1  "GearSelLck_D_Rq"
  PrkBrkActv_D_RqTrnGear/1 -> bus_creator/2  "PrkBrkActv_D_RqTrnGear"
  TrnCmdCnt_B_Actl/1 -> bus_creator/3  "TrnCmdCnt_B_Actl"
  TrnCmdState_B_Actl/1 -> bus_creator/4  "TrnCmdState_B_Actl"
  TrnDtpCmd_D_Actl/1 -> bus_creator/5  "TrnDtpCmd_D_Actl"
  TrnGearCmd_No_Cnt/1 -> bus_creator/6  "TrnGearCmd_No_Cnt"
  TrnGearCmd_No_Cs/1 -> bus_creator/7  "TrnGearCmd_No_Cs"
  TrnGearCmd_Pc_ActlPt/1 -> bus_creator/8  "TrnGearCmd_Pc_ActlPt"
  TrnGearMsgTxt_D_Rq/1 -> bus_creator/9  "TrnGearMsgTxt_D_Rq"
  TrnGearNtmAllow_B_Stat/1 -> bus_creator/10  "TrnGearNtmAllow_B_Stat"
  TrnGear_D_RqPt/1 -> bus_creator/11  "TrnGear_D_RqPt"
  TrnLvrV_D_Rq/1 -> bus_creator/12  "TrnLvrV_D_Rq"
  TrnNtrlTowCmd_D_Actl/1 -> bus_creator/13  "TrnNtrlTowCmd_D_Actl"
  TrnSbwSysHlth_D_Actl/1 -> bus_creator/14  "TrnSbwSysHlth_D_Actl"
  TrnValidGear_D_Cnfm/1 -> bus_creator/15  "TrnValidGear_D_Cnfm"

== system test_mdl/FD1_CAN_P702_GASD_MY21_DCV_V06/PCM/Global_PATS_TargetInfo ==
  bus_creator : BusCreator  Inputs=3
  immoTarget1Cmd : Constant
  immoTarget1Data : Constant
  immoTarget1Status : Constant
  port : Outport
  wires:
  bus_creator/1 -> port/1  "Global_PATS_TargetInfo"
  immoTarget1Cmd/1 -> bus_creator/1  "immoTarget1Cmd"
  immoTarget1Data/1 -> bus_creator/2  "immoTarget1Data"
  immoTarget1Status/1 -> bus_creator/3  "immoTarget1Status"

== system test_mdl/FD1_CAN_P702_GASD_MY21_DCV_V06/PCM/Low_Voltage_Power_Data_FD1 ==
  PwSrcULoComm_B_Falt : Constant
  PwSrcULoDcnnt_B_Stat : Constant
  PwSrcULoFalt_D_Stat : Constant
  PwSrcULoOvrTe_B_Actl : Constant
  PwSrcULo_I_Actl : Constant
  PwSrcULo_I_Mx : Constant
  PwSrcULo_Pc_Mx : Constant
  ULoRgenTestMde_B_Stat : Constant
  bus_creator : BusCreator  Inputs=8
  port : Outport
  wires:
  bus_creator/1 -> port/1  "Low_Voltage_Power_Data_FD1"
  PwSrcULoComm_B_Falt/1 -> bus_creator/1  "PwSrcULoComm_B_Falt"
  PwSrcULoDcnnt_B_Stat/1 -> bus_creator/2  "PwSrcULoDcnnt_B_Stat"
  PwSrcULoFalt_D_Stat/1 -> bus_creator/3  "PwSrcULoFalt_D_Stat"
  PwSrcULoOvrTe_B_Actl/1 -> bus_creator/4  "PwSrcULoOvrTe_B_Actl"
  PwSrcULo_I_Actl/1 -> bus_creator/5  "PwSrcULo_I_Actl"
  PwSrcULo_I_Mx/1 -> bus_creator/6  "PwSrcULo_I_Mx"
  PwSrcULo_Pc_Mx/1 -> bus_creator/7  "PwSrcULo_Pc_Mx"
  ULoRgenTestMde_B_Stat/1 -> bus_creator/8  "ULoRgenTestMde_B_Stat"

== system test_mdl/FD1_CAN_P702_GASD_MY21_DCV_V06/PCM/OTAPhysPCMtoGWM_ECG ==
  OTAPhysPCMtoGWM_ECG : Constant
  bus_creator : BusCreator  Inputs=1
  port : Outport
  wires:
  bus_creator/1 -> port/1  "OTAPhysPCMtoGWM_ECG"
  OTAPhysPCMtoGWM_ECG/1 -> bus_creator/1  "OTAPhysPCMtoGWM_ECG"

== system test_mdl/FD1_CAN_P702_GASD_MY21_DCV_V06/PCM/PARSEDPhysPCMtoGWM_ECG ==
  PARSEDPhysPCMtoGWM_ECG : Constant
  bus_creator : BusCreator  Inputs=1
  port : Outport
  wires:
  bus_creator/1 -> port/1  "PARSEDPhysPCMtoGWM_ECG"
  PARSEDPhysPCMtoGWM_ECG/1 -> bus_creator/1  "PARSEDPhysPCMtoGWM_ECG"

== system test_mdl/FD1_CAN_P702_GASD_MY21_DCV_V06/PCM/PARSEDPushPCMtoGWM_ECG ==
  PARSEDPushPCMtoGWM_ECG : Constant
  bus_creator : BusCreator  Inputs=1
  port : Outport
  wires:
  bus_creator/1 -> port/1  "PARSEDPushPCMtoGWM_ECG"
  PARSEDPushPCMtoGWM_ECG/1 -> bus_creator/1  "PARSEDPushPCMtoGWM_ECG"

== system test_mdl/FD1_CAN_P702_GASD_MY21_DCV_V06/PCM/PCM_AutoSar_NetworkMgmt ==
  PCM_AutoSarNMControl : Constant
  PCM_AutoSarNMNodeId : Constant
  PCM_AutoSarNMReserved{1..4} (4 alike) : Constant
  PCM_GWNMProxy : Constant
  PCM_GWOnBoardTester : Constant
  bus_creator : BusCreator  Inputs=8
  port : Outport
  wires:
  bus_creator/1 -> port/1  "PCM_AutoSar_NetworkMgmt"
  PCM_AutoSarNMControl/1 -> bus_creator/1  "PCM_AutoSarNMControl"
  PCM_AutoSarNMNodeId/1 -> bus_creator/2  "PCM_AutoSarNMNodeId"
  PCM_AutoSarNMReserved1/1 -> bus_creator/3  "PCM_AutoSarNMReserved1"
  PCM_AutoSarNMReserved2/1 -> bus_creator/4  "PCM_AutoSarNMReserved2"
  PCM_AutoSarNMReserved3/1 -> bus_creator/5  "PCM_AutoSarNMReserved3"
  PCM_AutoSarNMReserved4/1 -> bus_creator/6  "PCM_AutoSarNMReserved4"
  PCM_GWNMProxy/1 -> bus_creator/7  "PCM_GWNMProxy"
  PCM_GWOnBoardTester/1 -> bus_creator/8  "PCM_GWOnBoardTester"

== system test_mdl/FD1_CAN_P702_GASD_MY21_DCV_V06/PCM/PCM_Rapid_Data_Response_1 ==
  UUDTPCMResponse1 : Constant
  bus_creator : BusCreator  Inputs=1
  port : Outport
  wires:
  bus_creator/1 -> port/1  "PCM_Rapid_Data_Response_1"
  UUDTPCMResponse1/1 -> bus_creator/1  "UUDTPCMResponse1"

== system test_mdl/FD1_CAN_P702_GASD_MY21_DCV_V06/PCM/PCM_Rapid_Data_Response_2 ==
  UUDTPCMResponse2 : Constant
  bus_creator : BusCreator  Inputs=1
  port : Outport
  wires:
  bus_creator/1 -> port/1  "PCM_Rapid_Data_Response_2"
  UUDTPCMResponse2/1 -> bus_creator/1  "UUDTPCMResponse2"

== system test_mdl/FD1_CAN_P702_GASD_MY21_DCV_V06/PCM/PowertrainData_1 ==
  AirCondFluidHi_P_Actl : Constant
  CoolantFanStepAct : Constant
  ECMMILRequest : Constant
  EngIdlShutDown_D_Stat : Constant
  EngIdlShutDwnTxt_D_Rq : Constant
  FUEL_ALCOHOL_PERCNT : Constant
  FohEng_D_Rq : Constant
  OilPressureWarning : Constant
  TrnTotLss_Tq_Est : Constant
  TrnTotTq_Rt_Est : Constant
  VehVLimActv_B_Actl : Constant
  VehVLimStat_D_Actl : Constant
  bus_creator : BusCreator  Inputs=12
  port : Outport
  wires:
  bus_creator/1 -> port/1  "PowertrainData_1"
  AirCondFluidHi_P_Actl/1 -> bus_creator/1  "AirCondFluidHi_P_Actl"
  CoolantFanStepAct/1 -> bus_creator/2  "CoolantFanStepAct"
  ECMMILRequest/1 -> bus_creator/3  "ECMMILRequest"
  EngIdlShutDown_D_Stat/1 -> bus_creator/4  "EngIdlShutDown_D_Stat"
  EngIdlShutDwnTxt_D_Rq/1 -> bus_creator/5  "EngIdlShutDwnTxt_D_Rq"
  FUEL_ALCOHOL_PERCNT/1 -> bus_creator/6  "FUEL_ALCOHOL_PERCNT"
  FohEng_D_Rq/1 -> bus_creator/7  "FohEng_D_Rq"
  OilPressureWarning/1 -> bus_creator/8  "OilPressureWarning"
  TrnTotLss_Tq_Est/1 -> bus_creator/9  "TrnTotLss_Tq_Est"
  TrnTotTq_Rt_Est/1 -> bus_creator/10  "TrnTotTq_Rt_Est"
  VehVLimActv_B_Actl/1 -> bus_creator/11  "VehVLimActv_B_Actl"
  VehVLimStat_D_Actl/1 -> bus_creator/12  "VehVLimStat_D_Actl"

== system test_mdl/FD1_CAN_P702_GASD_MY21_DCV_V06/PCM/PowertrainData_10 ==
  GearEngag_D_Actl : Constant
  GearLvr_D_ActlDrv : Constant
  GearPos_D_Actl : Constant
  GearPos_D_Trg : Constant
  GearPos_No_Cnt : Constant
  GearPos_No_Cs : Constant
  TrnIgnOffDly_T_Rq : Constant
  TrnPrkSys_D_Actl : Constant
  TrnRng_D_Rq : Constant
  bus_creator : BusCreator  Inputs=9
  port : Outport
  wires:
  bus_creator/1 -> port/1  "PowertrainData_10"
  GearEngag_D_Actl/1 -> bus_creator/1  "GearEngag_D_Actl"
  GearLvr_D_ActlDrv/1 -> bus_creator/2  "GearLvr_D_ActlDrv"
  GearPos_D_Actl/1 -> bus_creator/3  "GearPos_D_Actl"
  GearPos_D_Trg/1 -> bus_creator/4  "GearPos_D_Trg"
  GearPos_No_Cnt/1 -> bus_creator/5  "GearPos_No_Cnt"
  GearPos_No_Cs/1 -> bus_creator/6  "GearPos_No_Cs"
  TrnIgnOffDly_T_Rq/1 -> bus_creator/7  "TrnIgnOffDly_T_Rq"
  TrnPrkSys_D_Actl/1 -> bus_creator/8  "TrnPrkSys_D_Actl"
  TrnRng_D_Rq/1 -> bus_creator/9  "TrnRng_D_Rq"

== system test_mdl/FD1_CAN_P702_GASD_MY21_DCV_V06/PCM/PowertrainData_2 ==
  ApedPos_Pc_ActlDiag : Constant
  EngAirIn_Te_Actl : Constant
  EngClnt_Te_ActlDiag : Constant
  EngLoad_Pc_CalcDiag : Constant
  EngMsgTxt_D_Rq : Constant
  GrllShtrPos_B_Falt : Constant
  GrllShtrPos_D_Cmd : Constant
  IsaOffst_D_Stat : Constant
  ObdWarmUp_B_Complt : Constant
  SlMde_D_RqDsply : Constant
  SlMde_D_Stat : Constant
  bus_creator : BusCreator  Inputs=11
  port : Outport
  wires:
  bus_creator/1 -> port/1  "PowertrainData_2"
  ApedPos_Pc_ActlDiag/1 -> bus_creator/1  "ApedPos_Pc_ActlDiag"
  EngAirIn_Te_Actl/1 -> bus_creator/2  "EngAirIn_Te_Actl"
  EngClnt_Te_ActlDiag/1 -> bus_creator/3  "EngClnt_Te_ActlDiag"
  EngLoad_Pc_CalcDiag/1 -> bus_creator/4  "EngLoad_Pc_CalcDiag"
  EngMsgTxt_D_Rq/1 -> bus_creator/5  "EngMsgTxt_D_Rq"
  GrllShtrPos_B_Falt/1 -> bus_creator/6  "GrllShtrPos_B_Falt"
  GrllShtrPos_D_Cmd/1 -> bus_creator/7  "GrllShtrPos_D_Cmd"
  IsaOffst_D_Stat/1 -> bus_creator/8  "IsaOffst_D_Stat"
  ObdWarmUp_B_Complt/1 -> bus_creator/9  "ObdWarmUp_B_Complt"
  SlMde_D_RqDsply/1 -> bus_creator/10  "SlMde_D_RqDsply"
  SlMde_D_Stat/1 -> bus_creator/11  "SlMde_D_Stat"

== system test_mdl/FD1_CAN_P702_GASD_MY21_DCV_V06/PCM/PowertrainData_3 ==
  BattULoChrg_U_Cmd : Constant
  ElLoadCtl_D_Rq : Constant
  EngMnfld_P_Actl : Constant
  FuelPumpPwr_B_Rq : Constant
  bus_creator : BusCreator  Inputs=4
  port : Outport
  wires:
  bus_creator/1 -> port/1  "PowertrainData_3"
  BattULoChrg_U_Cmd/1 -> bus_creator/1  "BattULoChrg_U_Cmd"
  ElLoadCtl_D_Rq/1 -> bus_creator/2  "ElLoadCtl_D_Rq"
  EngMnfld_P_Actl/1 -> bus_creator/3  "EngMnfld_P_Actl"
  FuelPumpPwr_B_Rq/1 -> bus_creator/4  "FuelPumpPwr_B_Rq"

== system test_mdl/FD1_CAN_P702_GASD_MY21_DCV_V06/PCM/PowertrainData_6 ==
  BrkTot_Tq_RqFapLc : Constant
  FapLc_B_Err : Constant
  TrnAin_Pc_RqDrv : Constant
  bus_creator : BusCreator  Inputs=3
  port : Outport
  wires:
  bus_creator/1 -> port/1  "PowertrainData_6"
  BrkTot_Tq_RqFapLc/1 -> bus_creator/1  "BrkTot_Tq_RqFapLc"
  FapLc_B_Err/1 -> bus_creator/2  "FapLc_B_Err"
  TrnAin_Pc_RqDrv/1 -> bus_creator/3  "TrnAin_Pc_RqDrv"

== system test_mdl/FD1_CAN_P702_GASD_MY21_DCV_V06/PCM/PowertrainData_7 ==
  EcoCochA_Pc_Dsply : Constant
  EcoCochCrus_Pc_Dsply : Constant
  EcoCochDecel_Pc_Dsply : Constant
  EcoCochIdlFuel_Pc_Dsply : Constant
  EcoCochInstNeg_B_Dsply : Constant
  EcoCochInst_Pc_Dsply : Constant
  EcoCochShif_Pc_Dsply : Constant
  bus_creator : BusCreator  Inputs=7
  port : Outport
  wires:
  bus_creator/1 -> port/1  "PowertrainData_7"
  EcoCochA_Pc_Dsply/1 -> bus_creator/1  "EcoCochA_Pc_Dsply"
  EcoCochCrus_Pc_Dsply/1 -> bus_creator/2  "EcoCochCrus_Pc_Dsply"
  EcoCochDecel_Pc_Dsply/1 -> bus_creator/3  "EcoCochDecel_Pc_Dsply"
  EcoCochIdlFuel_Pc_Dsply/1 -> bus_creator/4  "EcoCochIdlFuel_Pc_Dsply"
  EcoCochInstNeg_B_Dsply/1 -> bus_creator/5  "EcoCochInstNeg_B_Dsply"
  EcoCochInst_Pc_Dsply/1 -> bus_creator/6  "EcoCochInst_Pc_Dsply"
  EcoCochShif_Pc_Dsply/1 -> bus_creator/7  "EcoCochShif_Pc_Dsply"

== system test_mdl/FD1_CAN_P702_GASD_MY21_DCV_V06/PCM/PowertrainData_9 ==
  AutoTowActv_B_Stat : Constant
  AutoTowAllw_D_StatMnu : Constant
  EngExhMdeQuiet_D2_Stat : Constant
  GrossTrainWeight_M_Est : Constant
  HvacCmprLim_D_Stat : Constant
  TrailCtlPt_B_Falt : Constant
  Veh_V_DsplyTrailCtlSet : Constant
  WakeAlarm1_B_Typ : Constant
  WakeAlarm1_T_Rq : Constant
  bus_creator : BusCreator  Inputs=9
  port : Outport
  wires:
  bus_creator/1 -> port/1  "PowertrainData_9"
  AutoTowActv_B_Stat/1 -> bus_creator/1  "AutoTowActv_B_Stat"
  AutoTowAllw_D_StatMnu/1 -> bus_creator/2  "AutoTowAllw_D_StatMnu"
  EngExhMdeQuiet_D2_Stat/1 -> bus_creator/3  "EngExhMdeQuiet_D2_Stat"
  GrossTrainWeight_M_Est/1 -> bus_creator/4  "GrossTrainWeight_M_Est"
  HvacCmprLim_D_Stat/1 -> bus_creator/5  "HvacCmprLim_D_Stat"
  TrailCtlPt_B_Falt/1 -> bus_creator/6  "TrailCtlPt_B_Falt"
  Veh_V_DsplyTrailCtlSet/1 -> bus_creator/7  "Veh_V_DsplyTrailCtlSet"
  WakeAlarm1_B_Typ/1 -> bus_creator/8  "WakeAlarm1_B_Typ"
  WakeAlarm1_T_Rq/1 -> bus_creator/9  "WakeAlarm1_T_Rq"

== system test_mdl/FD1_CAN_P702_GASD_MY21_DCV_V06/PCM/Powertrain_Data_4 ==
  BpedDrvMsgTxt_B_Dsply : Constant
  FuelLvlWarn_D_ActlEng : Constant
  FuelLvl_Pc_DsplyEng : Constant
  FuelRange_L_DsplyEng : Constant
  RearDiffOilTeWarn_B_Rq : Constant
  RearDiffOil_Te_Actl : Constant
  SelDrvMdePt_D_Stat : Constant
  bus_creator : BusCreator  Inputs=7
  port : Outport
  wires:
  bus_creator/1 -> port/1  "Powertrain_Data_4"
  BpedDrvMsgTxt_B_Dsply/1 -> bus_creator/1  "BpedDrvMsgTxt_B_Dsply"
  FuelLvlWarn_D_ActlEng/1 -> bus_creator/2  "FuelLvlWarn_D_ActlEng"
  FuelLvl_Pc_DsplyEng/1 -> bus_creator/3  "FuelLvl_Pc_DsplyEng"
  FuelRange_L_DsplyEng/1 -> bus_creator/4  "FuelRange_L_DsplyEng"
  RearDiffOilTeWarn_B_Rq/1 -> bus_creator/5  "RearDiffOilTeWarn_B_Rq"
  RearDiffOil_Te_Actl/1 -> bus_creator/6  "RearDiffOil_Te_Actl"
  SelDrvMdePt_D_Stat/1 -> bus_creator/7  "SelDrvMdePt_D_Stat"

== system test_mdl/FD1_CAN_P702_GASD_MY21_DCV_V06/PCM/Powertrain_Data_5 ==
  AdasLcObtclAbrt_B_Stat : Constant
  AirDamPos_D_Stat : Constant
  BattRgenLoChrg_D_RqEng : Constant
  BattRgenLoDChrg_D_RqEng : Constant
  FapLcActv_B_Stat : Constant
  FapLcInhbt_B_Rq : Constant
  FapLcMaxGrdAbrt_B_Stat : Constant
  FapLcMaxGrdInhbt_B_Stat : Constant
  FapLcObstcl_B_Stat : Constant
  FapLcPrchgBrk_B_Rq : Constant
  FapLcStopHold_B_Rq : Constant
  bus_creator : BusCreator  Inputs=11
  port : Outport
  wires:
  bus_creator/1 -> port/1  "Powertrain_Data_5"
  AdasLcObtclAbrt_B_Stat/1 -> bus_creator/1  "AdasLcObtclAbrt_B_Stat"
  AirDamPos_D_Stat/1 -> bus_creator/2  "AirDamPos_D_Stat"
  BattRgenLoChrg_D_RqEng/1 -> bus_creator/3  "BattRgenLoChrg_D_RqEng"
  BattRgenLoDChrg_D_RqEng/1 -> bus_creator/4  "BattRgenLoDChrg_D_RqEng"
  FapLcActv_B_Stat/1 -> bus_creator/5  "FapLcActv_B_Stat"
  FapLcInhbt_B_Rq/1 -> bus_creator/6  "FapLcInhbt_B_Rq"
  FapLcMaxGrdAbrt_B_Stat/1 -> bus_creator/7  "FapLcMaxGrdAbrt_B_Stat"
  FapLcMaxGrdInhbt_B_Stat/1 -> bus_creator/8  "FapLcMaxGrdInhbt_B_Stat"
  FapLcObstcl_B_Stat/1 -> bus_creator/9  "FapLcObstcl_B_Stat"
  FapLcPrchgBrk_B_Rq/1 -> bus_creator/10  "FapLcPrchgBrk_B_Rq"
  FapLcStopHold_B_Rq/1 -> bus_creator/11  "FapLcStopHold_B_Rq"

== system test_mdl/FD1_CAN_P702_GASD_MY21_DCV_V06/PCM/Stop_Start ==
  AutoStopPtDelta_I_Est : Constant
  HiElPwInhbt_B_Stat : Constant
  OdoTripVerify_L_Actl : Constant
  StopStrtDrvMde_D_Indic : Constant
  StopStrtIODTxt_D_Rq : Constant
  StopStrtMsgTxt_D_Rq : Constant
  StopStrtStdby_D_Indic : Constant
  bus_creator : BusCreator  Inputs=7
  port : Outport
  wires:
  bus_creator/1 -> port/1  "Stop_Start"
  AutoStopPtDelta_I_Est/1 -> bus_creator/1  "AutoStopPtDelta_I_Est"
  HiElPwInhbt_B_Stat/1 -> bus_creator/2  "HiElPwInhbt_B_Stat"
  OdoTripVerify_L_Actl/1 -> bus_creator/3  "OdoTripVerify_L_Actl"
  StopStrtDrvMde_D_Indic/1 -> bus_creator/4  "StopStrtDrvMde_D_Indic"
  StopStrtIODTxt_D_Rq/1 -> bus_creator/5  "StopStrtIODTxt_D_Rq"
  StopStrtMsgTxt_D_Rq/1 -> bus_creator/6  "StopStrtMsgTxt_D_Rq"
  StopStrtStdby_D_Indic/1 -> bus_creator/7  "StopStrtStdby_D_Indic"

== system test_mdl/FD1_CAN_P702_GASD_MY21_DCV_V06/PCM/TesterPhysicalResPCM ==
  TesterPhysicalResPCM : Constant
  bus_creator : BusCreator  Inputs=1
  port : Outport
  wires:
  bus_creator/1 -> port/1  "TesterPhysicalResPCM"
  TesterPhysicalResPCM/1 -> bus_creator/1  "TesterPhysicalResPCM"

== system test_mdl/FD1_CAN_P702_GASD_MY21_DCV_V06/PCM/TorqueDataEngFlags ==
  PrplWhlTotTqRq_No_Cnt : Constant
  PrplWhlTotTqRq_No_Cs : Constant
  PrplWhlTot_Tq_LimMn : Constant
  PrplWhlTot_Tq_Rq : Constant
  PtDrvMde_D_Stat : Constant
  bus_creator : BusCreator  Inputs=5
  port : Outport
  wires:
  bus_creator/1 -> port/1  "TorqueDataEngFlags"
  PrplWhlTotTqRq_No_Cnt/1 -> bus_creator/1  "PrplWhlTotTqRq_No_Cnt"
  PrplWhlTotTqRq_No_Cs/1 -> bus_creator/2  "PrplWhlTotTqRq_No_Cs"
  PrplWhlTot_Tq_LimMn/1 -> bus_creator/3  "PrplWhlTot_Tq_LimMn"
  PrplWhlTot_Tq_Rq/1 -> bus_creator/4  "PrplWhlTot_Tq_Rq"
  PtDrvMde_D_Stat/1 -> bus_creator/5  "PtDrvMde_D_Stat"

== system test_mdl/FD1_CAN_P702_GASD_MY21_DCV_V06/PCM/TransGearData ==
  GboxOil_Te_Actl : Constant
  GearLvrPos_D_Actl : Constant
  SelDrvMdeSwtch_D_Stat3 : Constant
  TrnShifActv_B_Actl : Constant
  TrnSrvcRqd_B_Rq : Constant
  bus_creator : BusCreator  Inputs=5
  port : Outport
  wires:
  bus_creator/1 -> port/1  "TransGearData"
  GboxOil_Te_Actl/1 -> bus_creator/1  "GboxOil_Te_Actl"
  GearLvrPos_D_Actl/1 -> bus_creator/2  "GearLvrPos_D_Actl"
  SelDrvMdeSwtch_D_Stat3/1 -> bus_creator/3  "SelDrvMdeSwtch_D_Stat3"
  TrnShifActv_B_Actl/1 -> bus_creator/4  "TrnShifActv_B_Actl"
  TrnSrvcRqd_B_Rq/1 -> bus_creator/5  "TrnSrvcRqd_B_Rq"

== system test_mdl/FD1_CAN_P702_GASD_MY21_DCV_V06/PCM/VehicleOperatingModes ==
  ElPw_D_Stat : Constant
  ElPw_D_StatStrtStop : Constant
  Eng_D_Stat : Constant
  PlgActvArb_B_Actl : Constant
  PrplWhlRgenMn_Tq_Actl : Constant
  PrplWhlTot2_Tq_Actl : Constant
  PwPckTq_D_Stat : Constant
  TrnAinTq_D_Qf : Constant
  TrnAin_Tq_Actl : Constant
  bus_creator : BusCreator  Inputs=9
  port : Outport
  wires:
  bus_creator/1 -> port/1  "VehicleOperatingModes"
  ElPw_D_Stat/1 -> bus_creator/1  "ElPw_D_Stat"
  ElPw_D_StatStrtStop/1 -> bus_creator/2  "ElPw_D_StatStrtStop"
  Eng_D_Stat/1 -> bus_creator/3  "Eng_D_Stat"
  PlgActvArb_B_Actl/1 -> bus_creator/4  "PlgActvArb_B_Actl"
  PrplWhlRgenMn_Tq_Actl/1 -> bus_creator/5  "PrplWhlRgenMn_Tq_Actl"
  PrplWhlTot2_Tq_Actl/1 -> bus_creator/6  "PrplWhlTot2_Tq_Actl"
  PwPckTq_D_Stat/1 -> bus_creator/7  "PwPckTq_D_Stat"
  TrnAinTq_D_Qf/1 -> bus_creator/8  "TrnAinTq_D_Qf"
  TrnAin_Tq_Actl/1 -> bus_creator/9  "TrnAin_Tq_Actl"

== system test_mdl/FD1_CAN_P702_GASD_MY21_DCV_V06/PCM_HEV/Cluster_HEV_Data10_FD1 ==
  RngPerChrgAvg_L_Dsply : Constant
  bus_creator : BusCreator  Inputs=1
  port : Outport
  wires:
  bus_creator/1 -> port/1  "Cluster_HEV_Data10_FD1"
  RngPerChrgAvg_L_Dsply/1 -> bus_creator/1  "RngPerChrgAvg_L_Dsply"

== system test_mdl/FD1_CAN_P702_GASD_MY21_DCV_V06/PCM_HEV/Cluster_HEV_Data1_FD1 ==
  ChrgStat_D_Dsply : Constant
  RgenTrip_L_Dsply : Constant
  RgenTrip_Pc_Dsply : Constant
  bus_creator : BusCreator  Inputs=3
  port : Outport
  wires:
  bus_creator/1 -> port/1  "Cluster_HEV_Data1_FD1"
  ChrgStat_D_Dsply/1 -> bus_creator/1  "ChrgStat_D_Dsply"
  RgenTrip_L_Dsply/1 -> bus_creator/2  "RgenTrip_L_Dsply"
  RgenTrip_Pc_Dsply/1 -> bus_creator/3  "RgenTrip_Pc_Dsply"

== system test_mdl/FD1_CAN_P702_GASD_MY21_DCV_V06/PCM_HEV/Cluster_HEV_Data2 ==
  EffWhlLvl2_Pc_Dsply : Constant
  EffWhlThresOn_B_Dsply : Constant
  EffWhlThres_Pc_Dsply : Constant
  EngActv_B_Dsply : Constant
  EngOnMsg1_D_Dsply : Constant
  EngOnMsg2_D_Dsply : Constant
  EngPwLvl_Pc_Dsply : Constant
  FuelMaintMde_D_Dsply : Constant
  PwrFlowTxt_D_Dsply : Constant
  bus_creator : BusCreator  Inputs=9
  port : Outport
  wires:
  bus_creator/1 -> port/1  "Cluster_HEV_Data2"
  EffWhlLvl2_Pc_Dsply/1 -> bus_creator/1  "EffWhlLvl2_Pc_Dsply"
  EffWhlThresOn_B_Dsply/1 -> bus_creator/2  "EffWhlThresOn_B_Dsply"
  EffWhlThres_Pc_Dsply/1 -> bus_creator/3  "EffWhlThres_Pc_Dsply"
  EngActv_B_Dsply/1 -> bus_creator/4  "EngActv_B_Dsply"
  EngOnMsg1_D_Dsply/1 -> bus_creator/5  "EngOnMsg1_D_Dsply"
  EngOnMsg2_D_Dsply/1 -> bus_creator/6  "EngOnMsg2_D_Dsply"
  EngPwLvl_Pc_Dsply/1 -> bus_creator/7  "EngPwLvl_Pc_Dsply"
  FuelMaintMde_D_Dsply/1 -> bus_creator/8  "FuelMaintMde_D_Dsply"
  PwrFlowTxt_D_Dsply/1 -> bus_creator/9  "PwrFlowTxt_D_Dsply"

== system test_mdl/FD1_CAN_P702_GASD_MY21_DCV_V06/PCM_HEV/Cluster_HEV_Data3_FD1 ==
  EffRgenThres_Pc_Dsply : Constant
  EngMdeMsgTxt_D_Rq : Constant
  RngPerChrgInst_L_Dsply : Constant
  bus_creator : BusCreator  Inputs=3
  port : Outport
  wires:
  bus_creator/1 -> port/1  "Cluster_HEV_Data3_FD1"
  EffRgenThres_Pc_Dsply/1 -> bus_creator/1  "EffRgenThres_Pc_Dsply"
  EngMdeMsgTxt_D_Rq/1 -> bus_creator/2  "EngMdeMsgTxt_D_Rq"
  RngPerChrgInst_L_Dsply/1 -> bus_creator/3  "RngPerChrgInst_L_Dsply"
